simulink model "untitled"  (R2022a)
settings: Solver=FixedStepDiscrete  StartTime=0.0  StopTime=10  RelTol=1e-3  EnableMultiTasking=on
PreLoadFcn:
  | test_init
InitFcn:
  | untitled
settings Model: Creator=HP  LastModifiedBy=HP
settings HardwareCC: ProdBitPerPointer=32  ProdBitPerSizeT=32  ProdBitPerPtrDiffT=32  ProdLargestAtomicFloat=None  ProdIntDivRoundTo=Undefined  ProdEndianess=Unspecified  ProdWordSize=32  ProdHWDeviceType=ASIC/FPGA->ASIC/FPGA  TargetBitPerPointer=64  TargetBitPerSizeT=64  TargetBitPerPtrDiffT=64  TargetLongLongMode=on  TargetIntDivRoundTo=Zero  TargetEndianess=LittleEndian  TargetWordSize=64  TargetHWDeviceType=Custom Processor->MATLAB Host Computer  ProdEqTarget=off

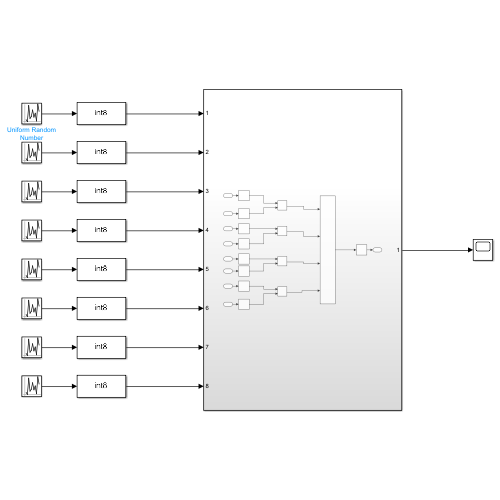
[thumbnail: Simulink's stored preview of the top-level diagram]
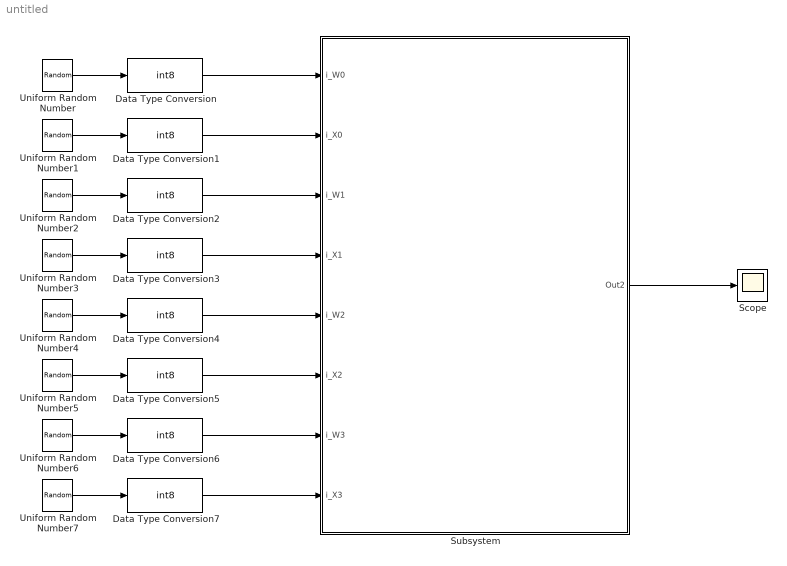
== system untitled ==
  Data Type Conversion{,1..7} (8 alike) : DataTypeConversion  OutDataTypeStr=int8  RndMeth=Round  SaturateOnIntegerOverflow=off
  Scope : Scope
  Subsystem : Subsystem
  Uniform Random Number : UniformRandomNumber  Minimum=0  Maximum=2^8-1  Seed=1  SampleTime=1
  Uniform Random Number1 : UniformRandomNumber  Minimum=0  Maximum=2^8-1  Seed=2  SampleTime=1
  Uniform Random Number2 : UniformRandomNumber  Minimum=0  Maximum=2^8-1  Seed=3  SampleTime=1
  Uniform Random Number3 : UniformRandomNumber  Minimum=0  Maximum=2^8-1  Seed=4  SampleTime=1
  Uniform Random Number4 : UniformRandomNumber  Minimum=0  Maximum=2^8-1  Seed=5  SampleTime=1
  Uniform Random Number5 : UniformRandomNumber  Minimum=0  Maximum=2^8-1  Seed=6  SampleTime=1
  Uniform Random Number6 : UniformRandomNumber  Minimum=0  Maximum=2^8-1  Seed=7  SampleTime=1
  Uniform Random Number7 : UniformRandomNumber  Minimum=0  Maximum=2^8-1  Seed=8  SampleTime=1
  wires:
  Uniform Random Number/1 -> Data Type Conversion/1
  Uniform Random Number1/1 -> Data Type Conversion1/1
  Uniform Random Number2/1 -> Data Type Conversion2/1
  Uniform Random Number3/1 -> Data Type Conversion3/1
  Uniform Random Number4/1 -> Data Type Conversion4/1
  Uniform Random Number5/1 -> Data Type Conversion5/1
  Uniform Random Number6/1 -> Data Type Conversion6/1
  Uniform Random Number7/1 -> Data Type Conversion7/1
  Data Type Conversion/1 -> Subsystem/1(i_W0)
  Data Type Conversion1/1 -> Subsystem/2(i_X0)
  Data Type Conversion2/1 -> Subsystem/3(i_W1)
  Data Type Conversion3/1 -> Subsystem/4(i_X1)
  Data Type Conversion4/1 -> Subsystem/5(i_W2)
  Data Type Conversion5/1 -> Subsystem/6(i_X2)
  Data Type Conversion6/1 -> Subsystem/7(i_W3)
  Data Type Conversion7/1 -> Subsystem/8(i_X3)
  Subsystem/1(Out2) -> Scope/1

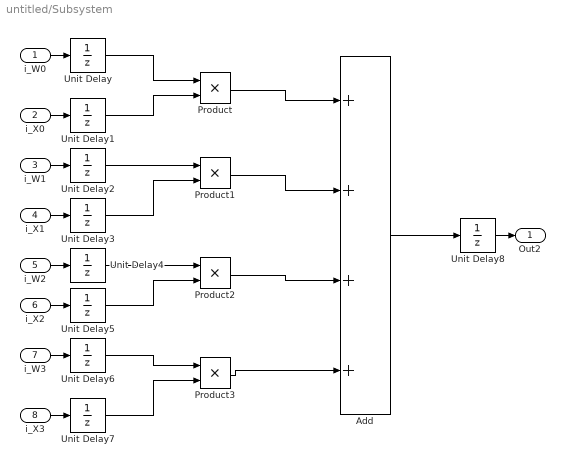
== system untitled/Subsystem ==
  i_W0 : Inport
  i_X0 : Inport  Port=2
  i_W1 : Inport  Port=3
  i_X1 : Inport  Port=4
  i_W2 : Inport  Port=5
  i_X2 : Inport  Port=6
  i_W3 : Inport  Port=7
  i_X3 : Inport  Port=8
  Add : Sum  Inputs=++++
  Product{,1..3} (4 alike) : Product
  Unit Delay{,1..8} (9 alike) : UnitDelay  SampleTime=-1  HasFrameUpgradeWarning=on
  Out2 : Outport
  wires:
  i_X2/1 -> Unit Delay5/1
  Product1/1 -> Add/2
  Unit Delay6/1 -> Product3/1
  Unit Delay7/1 -> Product3/2
  Unit Delay5/1 -> Product2/2
  Product/1 -> Add/1
  Unit Delay1/1 -> Product/2
  Unit Delay/1 -> Product/1
  Unit Delay4/1 -> Product2/1
  Unit Delay2/1 -> Product1/1
  Add/1 -> Unit Delay8/1
  Unit Delay3/1 -> Product1/2
  Product2/1 -> Add/3
  Product3/1 -> Add/4
  i_W2/1 -> Unit Delay4/1
  i_W3/1 -> Unit Delay6/1
  Unit Delay8/1 -> Out2/1
  i_W0/1 -> Unit Delay/1
  i_X0/1 -> Unit Delay1/1
  i_X3/1 -> Unit Delay7/1
  i_W1/1 -> Unit Delay2/1
  i_X1/1 -> Unit Delay3/1
